simulink model "LQG_tw"  (R2019a)
settings: Solver=FixedStepAuto  StartTime=0.0  StopTime=10  FixedStep=0.01  RelTol=1e-3
libraries: simulink x2
settings Model: Creator=chute  LastModifiedBy=chute

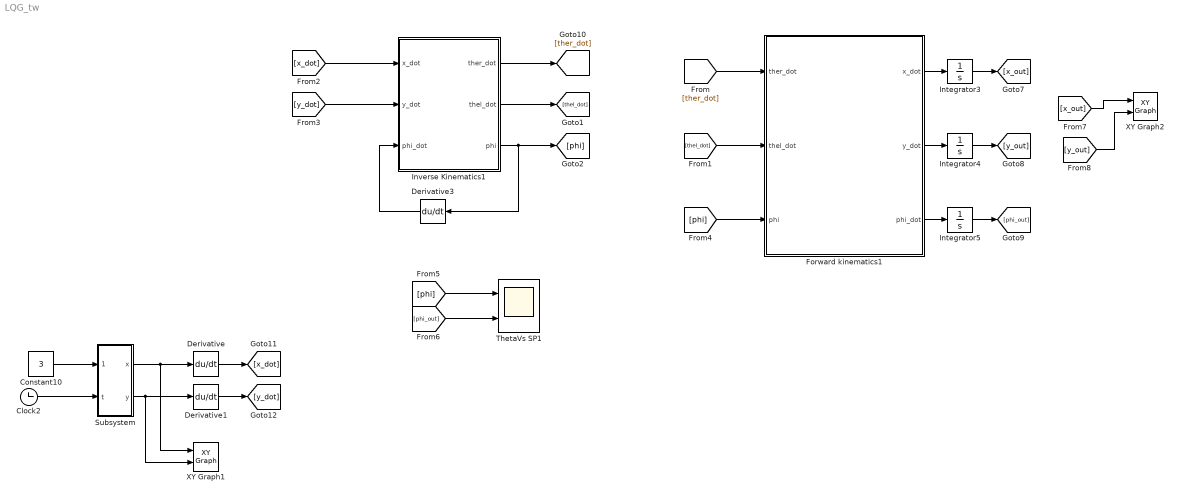
== system LQG_tw ==
  Clock2 : Clock
  Constant10 : Constant  Value=3
  Derivative : Derivative
  Derivative1 : Derivative
  Derivative3 : Derivative
  Forward kinematics1 : MATLAB Function  TreatAsAtomicUnit=on
  Integrator3 : Integrator
  Integrator4 : Integrator
  Integrator5 : Integrator  InitialCondition=[0;0]
  Inverse Kinematics1 : MATLAB Function  TreatAsAtomicUnit=on
  Subsystem : Subsystem
  ThetaVs SP1 : Scope  NumInputPorts=2
  XY Graph1 : simulink/Sinks/XY Graph  xmin=-1  xmax=1  ymin=-1  ymax=1  st=-1
  XY Graph2 : simulink/Sinks/XY Graph  xmin=-1  xmax=1  ymin=-1  ymax=1  st=-1
  wires:
  Forward kinematics1/2(y_dot) -> Integrator4/1
  Forward kinematics1/3(phi_dot) -> Integrator5/1
  [x_dot] -> Inverse Kinematics1/1(x_dot)
  Integrator4/1 -> [y_out]
  Integrator3/1 -> [x_out]
  Inverse Kinematics1/1(ther_dot) -> [ther_dot]
  Integrator5/1 -> [phi_out]
  Forward kinematics1/1(x_dot) -> Integrator3/1
  Inverse Kinematics1/2(thel_dot) -> [thel_dot]
  [y_dot] -> Inverse Kinematics1/2(y_dot)
  Subsystem/2(y) -> XY Graph1/2, Derivative1/1
  Clock2/1 -> Subsystem/2(t)
  Constant10/1 -> Subsystem/1(mode)
  Derivative1/1 -> [y_dot]
  Subsystem/1(x) -> Derivative/1, XY Graph1/1
  Derivative/1 -> [x_dot]
  [ther_dot] -> Forward kinematics1/1(ther_dot)
  [thel_dot] -> Forward kinematics1/2(thel_dot)
  [phi] -> ThetaVs SP1/1
  [phi_out] -> ThetaVs SP1/2
  [y_out] -> XY Graph2/2
  [x_out] -> XY Graph2/1
  Derivative3/1 -> Inverse Kinematics1/3(phi_dot)
  [phi] -> Forward kinematics1/3(phi)
  Inverse Kinematics1/3(phi) -> Derivative3/1, [phi]

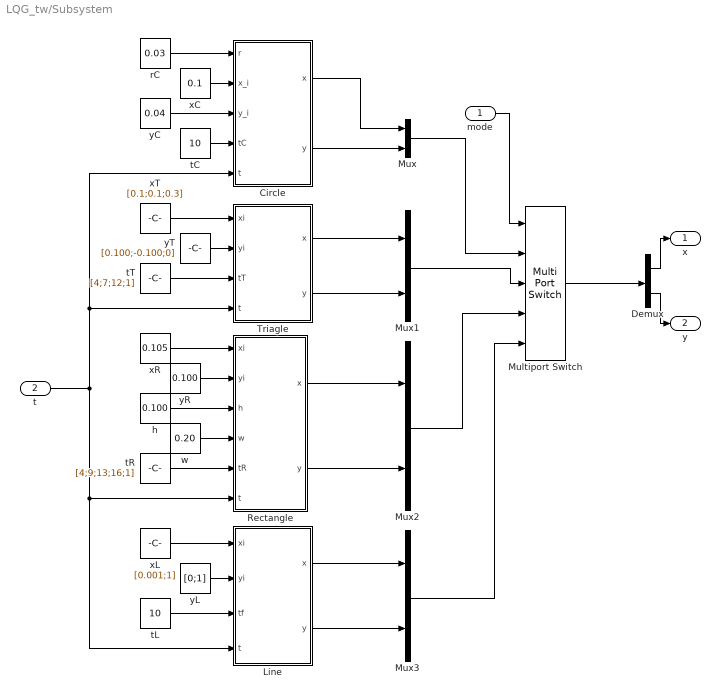
== system LQG_tw/Subsystem ==
  mode : Inport
  t : Inport  Port=2
  Circle : MATLAB Function  TreatAsAtomicUnit=on
  Demux : Demux  Outputs=2
  Line : MATLAB Function  TreatAsAtomicUnit=on
  Multiport Switch : MultiPortSwitch  DataPortOrder=Zero-based contiguous  Inputs=4  zeroidx=on
  Mux{,1..3} (4 alike) : Mux  Inputs=2
  Rectangle : MATLAB Function  TreatAsAtomicUnit=on
  Triagle : MATLAB Function  TreatAsAtomicUnit=on
  h : Constant  Value=0.100
  rC : Constant  Value=0.03
  tC : Constant  Value=10
  tL : Constant  Value=10
  tR : Constant  Value=[4;9;13;16;1]
  tT : Constant  Value=[4;7;12;1]
  w : Constant  Value=0.20
  xC : Constant  Value=0.1
  xL : Constant  Value=[0.001;1]
  xR : Constant  Value=0.105
  xT : Constant  Value=[0.1;0.1;0.3]
  yC : Constant  Value=0.04
  yL : Constant  Value=[0;1]
  yR : Constant  Value=0.100
  yT : Constant  Value=[0.100;-0.100;0]
  x : Outport
  y : Outport  Port=2
  wires:
  tR/1 -> Rectangle/5(tR)
  xL/1 -> Line/1(xi)
  Line/1(x) -> Mux3/1
  tC/1 -> Circle/4(tC)
  yL/1 -> Line/2(yi)
  tT/1 -> Triagle/3(tT)
  Multiport Switch/1 -> Demux/1
  Line/2(y) -> Mux3/2
  Triagle/1(x) -> Mux1/1
  Mux3/1 -> Multiport Switch/5
  xR/1 -> Rectangle/1(xi)
  Circle/2(y) -> Mux/2
  tL/1 -> Line/3(tf)
  w/1 -> Rectangle/4(w)
  Mux2/1 -> Multiport Switch/4
  mode/1 -> Multiport Switch/1
  Circle/1(x) -> Mux/1
  Mux1/1 -> Multiport Switch/3
  rC/1 -> Circle/1(r)
  Mux/1 -> Multiport Switch/2
  h/1 -> Rectangle/3(h)
  t/1 -> Circle/5(t), Triagle/4(t), Rectangle/6(t), Line/4(t)
  Demux/1 -> x/1
  xT/1 -> Triagle/1(xi)
  Rectangle/1(x) -> Mux2/1
  yT/1 -> Triagle/2(yi)
  xC/1 -> Circle/2(x_i)
  Triagle/2(y) -> Mux1/2
  yR/1 -> Rectangle/2(yi)
  Demux/2 -> y/1
  Rectangle/2(y) -> Mux2/2
  yC/1 -> Circle/3(y_i)

== matlab function LQG_tw/Forward kinematics1 ==
  data: ther_dot input; x_dot output; thel_dot input; y_dot output; phi_dot output; phi input
function [x_dot,y_dot,phi_dot] = FK(ther_dot,thel_dot,phi)
R =0.0335; % Wheel radius
W =0.17; % Body width
% thel_dot= (the_dot-(phi_dot*W)/R);
% ther_dot= the_dot+phi_dot*W/(2*R);
for i=1:2
    J=[(R/2)*cos(phi(i)),(R/2)*cos(phi(i));
       (R/2)*sin(phi(i)),(R/2)*sin(phi(i));
                     R/W,           -R/W];
end
out =J*[ther_dot;thel_dot];
x_dot=out(1,1);
y_dot =out(2,1);
phi_dot=out(3,1);
end

== matlab function LQG_tw/Inverse Kinematics1 ==
  data: x_dot input; ther_dot output; y_dot input; phi_dot input; thel_dot output; phi output
function [ther_dot,thel_dot,phi] = fcn(x_dot,y_dot,phi_dot)

R =0.0335; % Wheel radius
W =0.17; % Body width
a=y_dot;
b=-x_dot;
d=0;
anp = atan2(b, a);
x1 = anp + atan2(sqrt(a*a + b*b - d*d), d);
x2 = anp + atan2(-sqrt(a*a + b*b - d*d), d);
phi=[x1;x2];
    for i=1:2
        j=(1/R)*[cos(phi(i)),sin(phi(i)),W/(2);
                 cos(phi(i)),sin(phi(i)),-W/(2)];
        out1=j*[x_dot;y_dot;phi_dot(i)];
    end
ther_dot=out1(1,1);
thel_dot=out1(2,1);

== matlab function LQG_tw/Subsystem/Circle ==
  data: x output; r input; x_i input; y_i input; tC input; y output; t input
% Circle
function [x,y] = fcn(r,x_i,y_i,tC,t)
t0 = 3;
if (t-t0) <=tC
    x = x_i + r*cos(2*pi*(t-t0)/tC);
    y = y_i + r*sin(2*pi*(t-t0)/tC);
else
    x = x_i + r*cos(2*pi);
    y = y_i + r*sin(2*pi);
end

== matlab function LQG_tw/Subsystem/Line ==
  data: x output; xi input; yi input; tf input; y output; t input
% Triangle
function [x,y] = fcn(xi,yi,tf,t)
A = [xi(1);yi(1)];
B = [xi(2);yi(2)];
v0 = [0;0];
vf = [0;0];
t0=0;
if t<=tf
    Y = transpose([A v0 B vf]);
    K = [1 t0 t0^2 t0^3;
         0  1 2*t0 3*t0^2;
         1 tf tf^2 tf^3;
         0  1 2*tf 3*tf^2];
    X = inv(K)*Y;
    a = transpose(X);
    x = a(1,1) + a(1,2)*t + a(1,3)*t^2 + a(1,4)*t^3;

    y = a(2,1) + a(2,2)*t + a(2,3)*t^2 + a(2,4)*t^3;
else
    x = B(1);
    y = B(2);
end

== matlab function LQG_tw/Subsystem/Rectangle ==
  data: x output; xi input; yi input; h input; w input; tR input; y output; t input
% rectangle
function [x,y] = fcn(xi,yi,h,w,tR,t)
x1 = xi;
x2 = xi + w;
x3 = x2;
x4 = x1;
y1 = yi;
y2 = y1;
y3 = yi - h;
y4 = y3;
A = [x1;y1];
B = [x2;y2];
C = [x3;y3];
D = [x4;y4];
v0 = [0;0];
vf = [0;0];
t0=0;t1=tR(1);t2=tR(2);t3=tR(3);tf=tR(4);
td = tR(5);
td1 = t1+td;
td2 = t2+td;
td3 = t3+td;
if t<=t1
    Y = transpose([A v0 B vf]);
    K = [1 t0 t0^2 t0^3;
         0  1 2*t0 3*t0^2;
         1 t1 t1^2 t1^3;
         0  1 2*t1 3*t1^2];
    X = inv(K)*Y;
    a = transpose(X);
    x = a(1,1) + a(1,2)*t + a(1,3)*t^2 + a(1,4)*t^3;

    y = a(2,1) + a(2,2)*t + a(2,3)*t^2 + a(2,4)*t^3;
elseif (t>t1) && (t<=td1)
    x = B(1);y = B(2);
elseif (t>td1) && (t<=t2)
    Y = transpose([B v0 C vf]);
    K = [1 td1 td1^2 td1^3;
         0  1 2*td1 3*td1^2;
         1 t2 t2^2 t2^3;
         0  1 2*t2 3*t2^2];
    X = inv(K)*Y;
    a = transpose(X);
    x = a(1,1) + a(1,2)*t + a(1,3)*t^2 + a(1,4)*t^3;

    y = a(2,1) + a(2,2)*t + a(2,3)*t^2 + a(2,4)*t^3;
elseif (t>t2) && (t<=td2)
    x = C(1);y = C(2);
elseif (t>td2) && (t<=t3)
    Y = transpose([C v0 D vf]);
    K = [1 td2 td2^2 td2^3;
         0  1 2*td2 3*td2^2;
         1 t3 t3^2 t3^3;
         0  1 2*t3 3*t3^2];
    X = inv(K)*Y;
    a = transpose(X);
    x = a(1,1) + a(1,2)*t + a(1,3)*t^2 + a(1,4)*t^3;

    y = a(2,1) + a(2,2)*t + a(2,3)*t^2 + a(2,4)*t^3;
elseif (t>t3) && (t<=td3)
    x = D(1);y = D(2);
elseif (t>td3) && (t<=tf)
    Y = transpose([D v0 A vf]);
    K = [1 td3 td3^2 td3^3;
         0  1 2*td3 3*td3^2;
         1 tf tf^2 tf^3;
         0  1 2*tf 3*tf^2];
    X = inv(K)*Y;
    a = transpose(X);
    x = a(1,1) + a(1,2)*t + a(1,3)*t^2 + a(1,4)*t^3;

    y = a(2,1) + a(2,2)*t + a(2,3)*t^2 + a(2,4)*t^3;
else
    x = A(1);
    y = A(2);
end

== matlab function LQG_tw/Subsystem/Triagle ==
  data: x output; xi input; yi input; tT input; y output; t input
% Triangle
function [x,y] = fcn(xi,yi,tT,t)
A = [xi(1);yi(1)];
B = [xi(2);yi(2)];
C = [xi(3);yi(3)];
v0 = [0;0];
vf = [0;0];
t0=0;t1=tT(1);t2=tT(2);tf=tT(3);td = tT(1) + tT(4); tdd = tT(2) + tT(4);
if t<=t1
    Y = transpose([A v0 B vf]);
    K = [1 t0 t0^2 t0^3;
         0  1 2*t0 3*t0^2;
         1 t1 t1^2 t1^3;
         0  1 2*t1 3*t1^2];
    X = inv(K)*Y;
    a = transpose(X);
    x = a(1,1) + a(1,2)*t + a(1,3)*t^2 + a(1,4)*t^3;

    y = a(2,1) + a(2,2)*t + a(2,3)*t^2 + a(2,4)*t^3;
elseif (t>t1) && (t<=td)
    x = B(1);y = B(2);
elseif (t>td) && (t<=t2)
    Y = transpose([B v0 C vf]);
    K = [1 td td^2 td^3;
         0  1 2*td 3*td^2;
         1 t2 t2^2 t2^3;
         0  1 2*t2 3*t2^2];
    X = inv(K)*Y;
    a = transpose(X);
    x = a(1,1) + a(1,2)*t + a(1,3)*t^2 + a(1,4)*t^3;

    y = a(2,1) + a(2,2)*t + a(2,3)*t^2 + a(2,4)*t^3;
elseif (t>t2) && (t<=tdd)
    x = C(1);y = C(2);
elseif (t>tdd) && (t<=tf)
    Y = transpose([C v0 A vf]);
    K = [1 tdd tdd^2 tdd^3;
         0  1 2*tdd 3*tdd^2;
         1 tf tf^2 tf^3;
         0  1 2*tf 3*tf^2];
    X = inv(K)*Y;
    a = transpose(X);
    x = a(1,1) + a(1,2)*t + a(1,3)*t^2 + a(1,4)*t^3;

    y = a(2,1) + a(2,2)*t + a(2,3)*t^2 + a(2,4)*t^3;
else
    x = A(1);y = A(2);
end
